simulink model "mechanics_sensor"  (R2014a)
settings: Solver=ode45  StartTime=0.0  StopTime=10.0  RelTol=1e-3
values from neighbouring files (symbols this model uses):
  c = [x y z]'    [estimation_initfcn.m]
  I_xx = 1/12*m*(y^2+z^2)    (= 0.00181666666667)    [estimation_initfcn.m]
  I_yy = 1/12*m*(x^2+z^2)    (= 0.0418166666667)    [estimation_initfcn.m]
  I_zz = 1/12*m*(y^2+x^2)    (= 0.0433333333333)    [estimation_initfcn.m]
  m = 2    [estimation_initfcn.m]
  x = 0.5    [estimation_initfcn.m]
  y = 0.1    [estimation_initfcn.m]
  z = 0.03    [estimation_initfcn.m]
undefined symbols (not defined in the file or in its folder): X, Y, Z
libraries: nesl_utility x53, sm_lib x11, aerolibutil x6
settings Model: Creator=wirnshofer  LastModifiedBy=wirnshofer

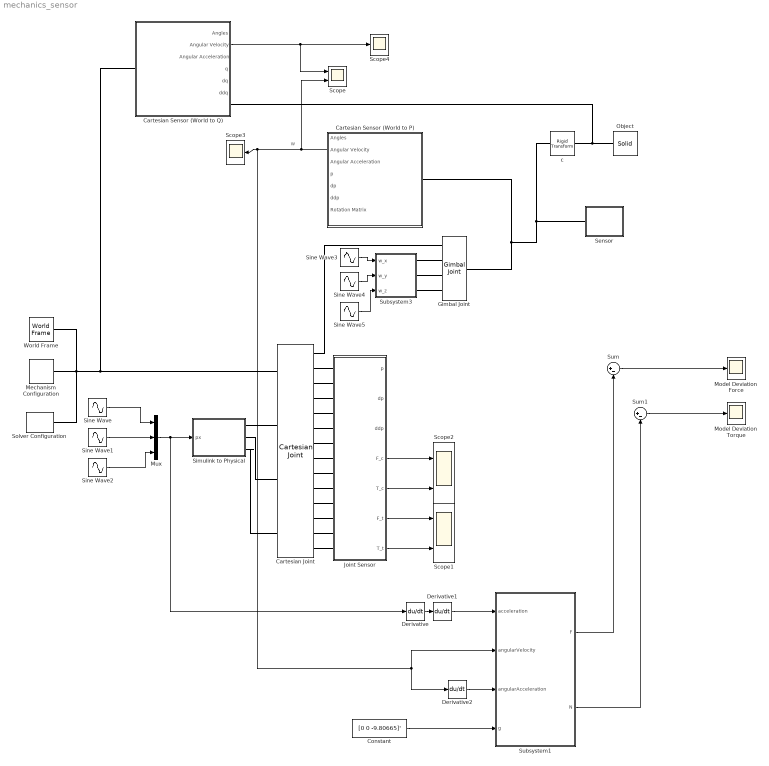
== system mechanics_sensor ==
  note: w
  Cartesian Joint : sm_lib/Joints/Cartesian Joint  SenseConstraintForce=on  SenseConstraintForceX=off  SenseConstraintForceY=off  SenseConstraintForceZ=off  SenseConstraintTorque=on  SenseConstraintTorqueX=off  SenseConstraintTorqueY=off  SenseConstraintTorqueZ=off  SenseTotalForce=on  SenseTotalForceX=off  SenseTotalForceY=off  SenseTotalForceZ=off  SenseTotalTorque=on  SenseTotalTorqueX=off  SenseTotalTorqueY=off  SenseTotalTorqueZ=off  CompositeWrenchDir=FollowerOnBase  CompositeWrenchFrame=BaseFrame  PxEquilibriumPosition=0  PxEquilibriumPositionUnits=m  PxSpringStiffness=0  PxSpringStiffnessUnits=N/m  PxDampingCoefficient=0  PxDampingCoefficientUnits=N/(m/s)  PxTorqueActuationMode=ComputedTorque  PxMotionActuationMode=InputMotion  PxSensePosition=on  PxSenseVelocity=on  PxSenseAcceleration=on  PxSenseTorqueForce=off  PxPositionTargetValue=0  PxPositionTargetValueUnits=m  PxPositionTargetSpecify=off  PxPositionTargetPriority=High  PxVelocityTargetValue=0  PxVelocityTargetValueUnits=m/s  PxVelocityTargetSpecify=off  PxVelocityTargetPriority=High  PyEquilibriumPosition=0  PyEquilibriumPositionUnits=m  PySpringStiffness=0  PySpringStiffnessUnits=N/m  PyDampingCoefficient=0  PyDampingCoefficientUnits=N/(m/s)  PyTorqueActuationMode=ComputedTorque  PyMotionActuationMode=InputMotion  PySensePosition=on  PySenseVelocity=on  PySenseAcceleration=on  PySenseTorqueForce=off  PyPositionTargetValue=0  PyPositionTargetValueUnits=m  PyPositionTargetSpecify=off  PyPositionTargetPriority=High  PyVelocityTargetValue=0  PyVelocityTargetValueUnits=m/s  PyVelocityTargetSpecify=off  PyVelocityTargetPriority=High  PzEquilibriumPosition=0  PzEquilibriumPositionUnits=m  PzSpringStiffness=0  PzSpringStiffnessUnits=N/m  PzDampingCoefficient=0  PzDampingCoefficientUnits=N/(m/s)  PzTorqueActuationMode=ComputedTorque  PzMotionActuationMode=InputMotion  PzSensePosition=on  PzSenseVelocity=on  PzSenseAcceleration=on  PzSenseTorqueForce=off  PzPositionTargetValue=0  PzPositionTargetValueUnits=m  PzPositionTargetSpecify=off  PzPositionTargetPriority=High  PzVelocityTargetValue=0  PzVelocityTargetValueUnits=m/s  PzVelocityTargetSpecify=off  PzVelocityTargetPriority=High  BlockFunction=simmechanics.library.joints.cartesian_joint
  Cartesian Sensor (World to P) : Subsystem
  Cartesian Sensor (World to Q) : Subsystem
  Constant : Constant  Value=[0 0 -9.80665]'
  Derivative : Derivative
  Derivative1 : Derivative
  Derivative2 : Derivative
  Gimbal Joint : sm_lib/Joints/Gimbal Joint  SenseConstraintForce=off  SenseConstraintForceX=off  SenseConstraintForceY=off  SenseConstraintForceZ=off  SenseConstraintTorque=off  SenseConstraintTorqueX=off  SenseConstraintTorqueY=off  SenseConstraintTorqueZ=off  SenseTotalForce=off  SenseTotalForceX=off  SenseTotalForceY=off  SenseTotalForceZ=off  SenseTotalTorque=off  SenseTotalTorqueX=off  SenseTotalTorqueY=off  SenseTotalTorqueZ=off  CompositeWrenchDir=FollowerOnBase  CompositeWrenchFrame=BaseFrame  RxEquilibriumPosition=0  RxEquilibriumPositionUnits=deg  RxSpringStiffness=0  RxSpringStiffnessUnits=N*m/deg  RxDampingCoefficient=0  RxDampingCoefficientUnits=N*m/(deg/s)  RxTorqueActuationMode=ComputedTorque  RxMotionActuationMode=InputMotion  RxSensePosition=off  RxSenseVelocity=off  RxSenseAcceleration=off  RxSenseTorqueForce=off  RxPositionTargetValue=0  RxPositionTargetValueUnits=deg  RxPositionTargetSpecify=off  RxPositionTargetPriority=High  RxVelocityTargetValue=0  RxVelocityTargetValueUnits=deg/s  RxVelocityTargetSpecify=off  RxVelocityTargetPriority=High  RyEquilibriumPosition=0  RyEquilibriumPositionUnits=deg  RySpringStiffness=0  RySpringStiffnessUnits=N*m/deg  RyDampingCoefficient=0  RyDampingCoefficientUnits=N*m/(deg/s)  RyTorqueActuationMode=ComputedTorque  RyMotionActuationMode=InputMotion  RySensePosition=off  RySenseVelocity=off  RySenseAcceleration=off  RySenseTorqueForce=off  RyPositionTargetValue=0  RyPositionTargetValueUnits=deg  RyPositionTargetSpecify=off  RyPositionTargetPriority=High  RyVelocityTargetValue=0  RyVelocityTargetValueUnits=deg/s  RyVelocityTargetSpecify=off  RyVelocityTargetPriority=High  RzEquilibriumPosition=0  RzEquilibriumPositionUnits=deg  RzSpringStiffness=0  RzSpringStiffnessUnits=N*m/deg  RzDampingCoefficient=0  RzDampingCoefficientUnits=N*m/(deg/s)  RzTorqueActuationMode=ComputedTorque  RzMotionActuationMode=InputMotion  RzSensePosition=off  RzSenseVelocity=off  RzSenseAcceleration=off  RzSenseTorqueForce=off  RzPositionTargetValue=0  RzPositionTargetValueUnits=deg  RzPositionTargetSpecify=off  RzPositionTargetPriority=High  RzVelocityTargetValue=0  RzVelocityTargetValueUnits=deg/s  RzVelocityTargetSpecify=off  RzVelocityTargetPriority=High  BlockFunction=simmechanics.library.joints.gimbal_joint
  Joint Sensor : Subsystem
  Mechanism Configuration : sm_lib/Utilities/Mechanism Configuration  UniformGravity=Constant  GravityVector=[0 0 -9.80665]  GravityUnits=m/s^2  LinearizationDelta=0.001  BlockFunction=simmechanics.library.utilities.mechanism_configuration
  Model Deviation Force : Scope
      settings: TimeRange=10  YMin=-1.3  YMax=0.8  SaveName=modelDeviationForce
  Model Deviation Torque : Scope
      settings: TimeRange=10  YMin=-1.3  YMax=0.8  SaveName=modelDeviationForce1
  Mux : Mux  Inputs=3
  Object : sm_lib/Body Elements/Solid  InertiaType=Custom  Mass=m  MassUnits=kg  CenterOfMass=[0 0 0]  CenterOfMassUnits=m  MomentsOfInertia=[I_xx I_yy I_zz]  MomentsOfInertiaUnits=kg*m^2  ProductsOfInertia=[0 0 0]  ProductsOfInertiaUnits=kg*m^2  DensityBased=on  Density=1000  DensityUnits=kg/(m^3)  GraphicType=FromGeometry  MarkerShape=Sphere  MarkerSize=10  MarkerSizeUnits=m  GraphicVisPropType=SimpleVisualProperties  GraphicDiffuseColor=[0.5 0.5 0.5]  GraphicSpecularColor=[0.5 0.5 0.5 1.0]  GraphicAmbientColor=[0.15 0.15 0.15 1.0]  GraphicEmissiveColor=[0.0 0.0 0.0 1.0]  GraphicShininess=75  GraphicOpacity=1.0  GeometryShape=Brick  RectangleSize=[1 1]  RectangleSizeUnits=m  BrickDimensions=[x y z]  BrickDimensionUnits=m  CylinderRadius=1  CylinderRadiusUnits=m  CylinderLength=1  CylinderLengthUnits=m  SphereRadius=1  SphereRadiusUnits=m  EllipsoidRadii=[1 1 1]  EllipsoidRadiiUnits=m  ExtrusionCrossSection=[1 1; -1 1; -1 -1; 1 -1]  ExtrusionCrossSectionUnits=m  ExtrusionLength=1  ExtrusionLengthUnits=m  PolygonNumSides=3  PolygonOuterRadius=1  PolygonOuterRadiusUnits=m  ExtGeomFileType=STL  ExtGeomFileUnits=m  RevolutionCrossSection=[1 1; 1 -1; 2 -1; 2 1]  RevolutionCrossSectionUnits=m  RevolutionExtent=Full  RevolutionAngle=180  RevolutionAngleUnits=deg  BlockFunction=simmechanics.library.body_elements.solid
  Scope : Scope  NumInputPorts=2
      settings: YMin=-0.3~-0.3  YMax=0.5~0.3
  Scope1 : Scope  NumInputPorts=2
      settings: TimeRange=10  YMin=-1.146992373051417~-500  YMax=1.739930939930119~500
  Scope2 : Scope  NumInputPorts=2
      settings: TimeRange=10  YMin=-1.146992373051417~-500  YMax=1.739930939930119~500  SaveName=ScopeData2
  Scope3 : Scope
      settings: YMin=-0.3  YMax=0.5  SaveName=ScopeData3
  Scope4 : Scope
      settings: YMin=-0.3  YMax=0.5  SaveName=ScopeData4
  Sensor : Subsystem
  Simulink to Physical : Subsystem
  Sine Wave : Sin  Amplitude=0.2  Frequency=7  SampleTime=0
  Sine Wave1 : Sin  Amplitude=0.3  Frequency=4  SampleTime=0
  Sine Wave2 : Sin  Amplitude=0.2  Frequency=10  SampleTime=0
  Sine Wave3 : Sin  Amplitude=0.5  Frequency=10  SampleTime=0
  Sine Wave4 : Sin  Amplitude=0.6  Frequency=8  SampleTime=0
  Sine Wave5 : Sin  Frequency=7  SampleTime=0
  Solver Configuration : nesl_utility/Solver Configuration  PhysicalDomain=network_engine_domain  SubClassName=solver  LeftPortType=input  RightPortType=generic  Accelerate=off  Tones=[]  Harmonics=[]  SimulateNoise=off  Profile=off  UseLocalSampling=off  EnableSwitchedLinearOptims=on  FrequencyDomain=off  UseCCode=off  RelTol=0.001  AbsTol=1e-06  MinStep=1e-09  ToWorkspace=off  DoDC=off  ResidualTolerance=1e-09  UseLocalSolver=off  LocalSolverChoice=NE_BACKWARD_EULER_ADVANCER  LocalSolverSampleTime=0.001  DoFixedCost=off  MaxNonlinIter=3  MaxModeIter=2  LinearAlgebra=Sparse  DelaysMemoryBudget=1024  AutomaticFiltering=on  FilteringTimeConstant=0.001
  Subsystem1 : Subsystem
  Subsystem3 : Subsystem
  Sum : Sum  Inputs=|+-
  Sum1 : Sum  Inputs=|+-
  World Frame : sm_lib/Frames and Transforms/World Frame  BlockFunction=simmechanics.library.frames_transforms.world_frame
  c : sm_lib/Frames and Transforms/Rigid Transform  TranslationMethod=Cartesian  TranslationLengthUnit=m  TranslationStandardAxis=+Z  TranslationStandardOffset=0  TranslationCartesianOffset=c  TranslationROffset=0  TranslationROffsetUnits=m  TranslationZOffset=0  TranslationZOffsetUnits=m  TranslationThetaOffset=0  TranslationThetaOffsetUnits=deg  RotationMethod=None  RotationAngleUnits=deg  RotationStandardAxis=+Z  RotationAngle=0  RotationArbitraryAxis=[0 0 1]  FollAlignAxisA=+X  BaseAlignAxisA=+Y  FollAlignAxisB=+Y  BaseAlignAxisB=+Z  BlockFunction=simmechanics.library.frames_transforms.rigid_transform
  wires:
  Sine Wave/1 -> Mux/1
  Sine Wave1/1 -> Mux/2
  Sine Wave2/1 -> Mux/3
  Joint Sensor/6(F_t) -> Scope1/1
  Joint Sensor/7(T_t) -> Scope1/2
  Joint Sensor/4(F_c) -> Scope2/1
  Joint Sensor/5(T_c) -> Scope2/2
  Cartesian Sensor (World to P)/2(Angular Velocity) -> Derivative2/1, Subsystem1/2(angularVelocity), Scope3/1, Scope/2
  Cartesian Sensor (World to Q)/2(Angular Velocity) -> Scope/1, Scope4/1
  Sine Wave3/1 -> Subsystem3/1(w_x)
  Sine Wave4/1 -> Subsystem3/2(w_y)
  Sine Wave5/1 -> Subsystem3/3(w_z)
  Mux/1 -> Derivative/1, Simulink to Physical/1(px)
  Derivative/1 -> Derivative1/1
  Derivative1/1 -> Subsystem1/1(acceleration)
  Derivative2/1 -> Subsystem1/3(angularAcceleration)
  Constant/1 -> Subsystem1/4(g)
  ? -> Sum/1
  Sum/1 -> Model Deviation Force/1
  ? -> Sum1/1
  Subsystem1/1(F) -> Sum/2
  Subsystem1/2(N) -> Sum1/2
  Sum1/1 -> Model Deviation Torque/1
  connections:
  Cartesian Sensor (World to Q)/RConn1 -- Object/RConn1 -- c/RConn1
  Solver Configuration/RConn1 -- World Frame/RConn1 -- Cartesian Joint/LConn1 -- Cartesian Sensor (World to Q)/LConn1 -- Mechanism Configuration/RConn1
  Gimbal Joint/RConn1 -- Cartesian Sensor (World to P)/LConn1 -- Sensor/RConn1 -- c/LConn1
  Simulink to Physical/RConn1 -- Cartesian Joint/LConn2
  Simulink to Physical/RConn2 -- Cartesian Joint/LConn3
  Simulink to Physical/RConn3 -- Cartesian Joint/LConn4
  Joint Sensor/LConn1 -- Cartesian Joint/RConn2
  Joint Sensor/LConn2 -- Cartesian Joint/RConn3
  Joint Sensor/LConn3 -- Cartesian Joint/RConn4
  Joint Sensor/LConn4 -- Cartesian Joint/RConn5
  Joint Sensor/LConn5 -- Cartesian Joint/RConn6
  Joint Sensor/LConn6 -- Cartesian Joint/RConn7
  Joint Sensor/LConn8 -- Cartesian Joint/RConn9
  Joint Sensor/LConn9 -- Cartesian Joint/RConn10
  Joint Sensor/LConn10 -- Cartesian Joint/RConn11
  Joint Sensor/LConn11 -- Cartesian Joint/RConn12
  Joint Sensor/LConn12 -- Cartesian Joint/RConn13
  Joint Sensor/LConn13 -- Cartesian Joint/RConn14
  Subsystem3/RConn1 -- Gimbal Joint/LConn2
  Subsystem3/RConn2 -- Gimbal Joint/LConn3
  Joint Sensor/LConn7 -- Cartesian Joint/RConn8
  Subsystem3/RConn3 -- Gimbal Joint/LConn4
  Cartesian Joint/RConn1 -- Gimbal Joint/LConn1

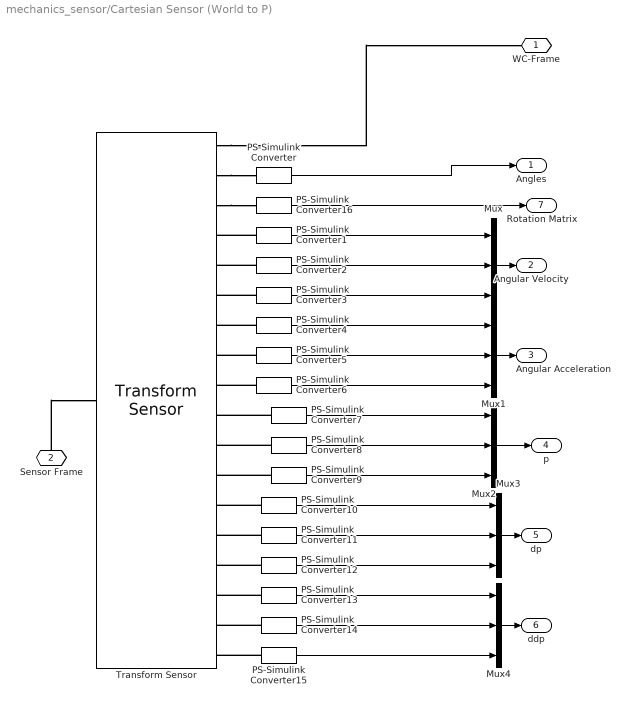
== system mechanics_sensor/Cartesian Sensor (World to P) ==
  Mux{,1..4} (5 alike) : Mux  Inputs=3
  PS-Simulink Converter{,1..16} (17 alike) : nesl_utility/PS-Simulink Converter  PhysicalDomain=network_engine_domain  SubClassName=ps_output  LeftPortType=input  RightPortType=output  PseudoPeriodic=off  Frequencies=[]  Unit=1  AffineConversion=off
  Transform Sensor : sm_lib/Frames and Transforms/Transform Sensor  MeasurementFrame=World  SenseAngle=on  SenseAxis=off  SenseAngle1=off  SenseAngle2=off  SenseAngle3=off  SenseQ=off  SenseR=on  SenseOmegaX=on  SenseOmegaY=on  SenseOmegaZ=on  SenseOmega1=off  SenseOmega2=off  SenseOmega3=off  SenseQDot=off  SenseRDot=off  SenseAlphaX=on  SenseAlphaY=on  SenseAlphaZ=on  SenseAlpha1=off  SenseAlpha2=off  SenseAlpha3=off  SenseQDDot=off  SenseRDDot=off  SenseX=on  SenseY=on  SenseZ=on  SenseRad=off  SenseAzim=off  SenseDist=off  SenseInc=off  SenseXDot=on  SenseYDot=on  SenseZDot=on  SenseRadDot=off  SenseAzimDot=off  SenseDistDot=off  SenseIncDot=off  SenseXDDot=on  SenseYDDot=on  SenseZDDot=on  SenseRadDDot=off  SenseAzimDDot=off  SenseDistDDot=off  SenseIncDDot=off  BlockFunction=simmechanics.library.frames_transforms.transform_sensor
  WC-Frame : PMIOPort  Port=1  Side=Right
  Sensor Frame : PMIOPort  Port=2  Side=Left
  Angles : Outport
  Angular Velocity : Outport  Port=2
  Angular Acceleration : Outport  Port=3
  p : Outport  Port=4
  dp : Outport  Port=5
  ddp : Outport  Port=6
  Rotation Matrix : Outport  Port=7
  wires:
  PS-Simulink Converter2/1 -> Mux/2
  PS-Simulink Converter5/1 -> Mux1/2
  Mux1/1 -> Angular Acceleration/1
  PS-Simulink Converter1/1 -> Mux/1
  Mux/1 -> Angular Velocity/1
  PS-Simulink Converter6/1 -> Mux1/3
  PS-Simulink Converter/1 -> Angles/1
  PS-Simulink Converter3/1 -> Mux/3
  PS-Simulink Converter4/1 -> Mux1/1
  PS-Simulink Converter8/1 -> Mux2/2
  Mux2/1 -> p/1
  PS-Simulink Converter9/1 -> Mux2/3
  PS-Simulink Converter7/1 -> Mux2/1
  PS-Simulink Converter11/1 -> Mux3/2
  Mux3/1 -> dp/1
  PS-Simulink Converter12/1 -> Mux3/3
  PS-Simulink Converter10/1 -> Mux3/1
  PS-Simulink Converter14/1 -> Mux4/2
  Mux4/1 -> ddp/1
  PS-Simulink Converter15/1 -> Mux4/3
  PS-Simulink Converter13/1 -> Mux4/1
  PS-Simulink Converter16/1 -> Rotation Matrix/1
  connections:
  Transform Sensor/RConn1 -- WC-Frame/RConn1
  Sensor Frame/RConn1 -- Transform Sensor/LConn1
  Transform Sensor/RConn2 -- PS-Simulink Converter/LConn1
  PS-Simulink Converter6/LConn1 -- Transform Sensor/RConn9
  PS-Simulink Converter2/LConn1 -- Transform Sensor/RConn5
  PS-Simulink Converter5/LConn1 -- Transform Sensor/RConn8
  PS-Simulink Converter1/LConn1 -- Transform Sensor/RConn4
  PS-Simulink Converter4/LConn1 -- Transform Sensor/RConn7
  PS-Simulink Converter3/LConn1 -- Transform Sensor/RConn6
  PS-Simulink Converter14/LConn1 -- Transform Sensor/RConn17
  PS-Simulink Converter10/LConn1 -- Transform Sensor/RConn13
  PS-Simulink Converter13/LConn1 -- Transform Sensor/RConn16
  PS-Simulink Converter12/LConn1 -- Transform Sensor/RConn15
  PS-Simulink Converter11/LConn1 -- Transform Sensor/RConn14
  PS-Simulink Converter15/LConn1 -- Transform Sensor/RConn18
  PS-Simulink Converter8/LConn1 -- Transform Sensor/RConn11
  PS-Simulink Converter9/LConn1 -- Transform Sensor/RConn12
  PS-Simulink Converter7/LConn1 -- Transform Sensor/RConn10
  Transform Sensor/RConn3 -- PS-Simulink Converter16/LConn1

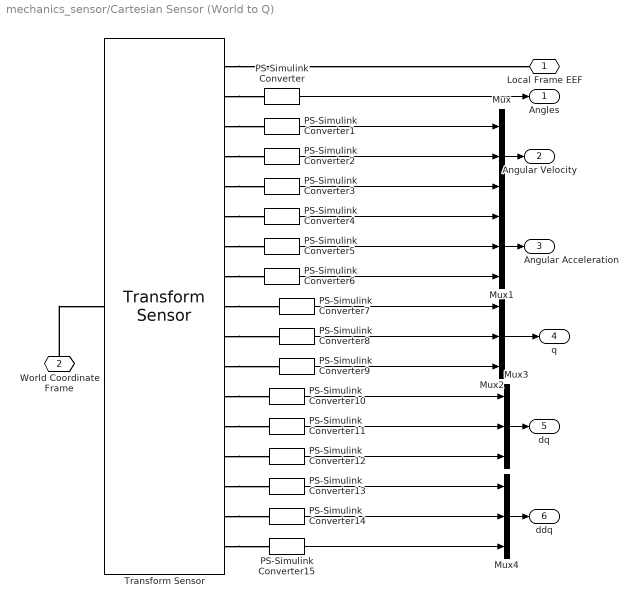
== system mechanics_sensor/Cartesian Sensor (World to Q) ==
  Mux{,1..4} (5 alike) : Mux  Inputs=3
  PS-Simulink Converter{,1..15} (16 alike) : nesl_utility/PS-Simulink Converter  PhysicalDomain=network_engine_domain  SubClassName=ps_output  LeftPortType=input  RightPortType=output  PseudoPeriodic=off  Frequencies=[]  Unit=1  AffineConversion=off
  Transform Sensor : sm_lib/Frames and Transforms/Transform Sensor  MeasurementFrame=World  SenseAngle=on  SenseAxis=off  SenseAngle1=off  SenseAngle2=off  SenseAngle3=off  SenseQ=off  SenseR=off  SenseOmegaX=on  SenseOmegaY=on  SenseOmegaZ=on  SenseOmega1=off  SenseOmega2=off  SenseOmega3=off  SenseQDot=off  SenseRDot=off  SenseAlphaX=on  SenseAlphaY=on  SenseAlphaZ=on  SenseAlpha1=off  SenseAlpha2=off  SenseAlpha3=off  SenseQDDot=off  SenseRDDot=off  SenseX=on  SenseY=on  SenseZ=on  SenseRad=off  SenseAzim=off  SenseDist=off  SenseInc=off  SenseXDot=on  SenseYDot=on  SenseZDot=on  SenseRadDot=off  SenseAzimDot=off  SenseDistDot=off  SenseIncDot=off  SenseXDDot=on  SenseYDDot=on  SenseZDDot=on  SenseRadDDot=off  SenseAzimDDot=off  SenseDistDDot=off  SenseIncDDot=off  BlockFunction=simmechanics.library.frames_transforms.transform_sensor
  Local Frame EEF : PMIOPort  Port=1  Side=Right
  World Coordinate Frame : PMIOPort  Port=2  Side=Left
  Angles : Outport
  Angular Velocity : Outport  Port=2
  Angular Acceleration : Outport  Port=3
  q : Outport  Port=4
  dq : Outport  Port=5
  ddq : Outport  Port=6
  wires:
  PS-Simulink Converter2/1 -> Mux/2
  PS-Simulink Converter5/1 -> Mux1/2
  Mux1/1 -> Angular Acceleration/1
  PS-Simulink Converter1/1 -> Mux/1
  Mux/1 -> Angular Velocity/1
  PS-Simulink Converter6/1 -> Mux1/3
  PS-Simulink Converter/1 -> Angles/1
  PS-Simulink Converter3/1 -> Mux/3
  PS-Simulink Converter4/1 -> Mux1/1
  PS-Simulink Converter8/1 -> Mux2/2
  Mux2/1 -> q/1
  PS-Simulink Converter9/1 -> Mux2/3
  PS-Simulink Converter7/1 -> Mux2/1
  PS-Simulink Converter11/1 -> Mux3/2
  Mux3/1 -> dq/1
  PS-Simulink Converter12/1 -> Mux3/3
  PS-Simulink Converter10/1 -> Mux3/1
  PS-Simulink Converter14/1 -> Mux4/2
  Mux4/1 -> ddq/1
  PS-Simulink Converter15/1 -> Mux4/3
  PS-Simulink Converter13/1 -> Mux4/1
  connections:
  Transform Sensor/RConn7 -- PS-Simulink Converter5/LConn1
  Transform Sensor/RConn1 -- Local Frame EEF/RConn1
  Transform Sensor/RConn5 -- PS-Simulink Converter3/LConn1
  Transform Sensor/RConn8 -- PS-Simulink Converter6/LConn1
  Transform Sensor/RConn3 -- PS-Simulink Converter1/LConn1
  Transform Sensor/RConn6 -- PS-Simulink Converter4/LConn1
  World Coordinate Frame/RConn1 -- Transform Sensor/LConn1
  Transform Sensor/RConn4 -- PS-Simulink Converter2/LConn1
  Transform Sensor/RConn2 -- PS-Simulink Converter/LConn1
  Transform Sensor/RConn9 -- PS-Simulink Converter7/LConn1
  Transform Sensor/RConn10 -- PS-Simulink Converter8/LConn1
  Transform Sensor/RConn11 -- PS-Simulink Converter9/LConn1
  Transform Sensor/RConn12 -- PS-Simulink Converter10/LConn1
  Transform Sensor/RConn13 -- PS-Simulink Converter11/LConn1
  Transform Sensor/RConn14 -- PS-Simulink Converter12/LConn1
  Transform Sensor/RConn15 -- PS-Simulink Converter13/LConn1
  Transform Sensor/RConn16 -- PS-Simulink Converter14/LConn1
  Transform Sensor/RConn17 -- PS-Simulink Converter15/LConn1

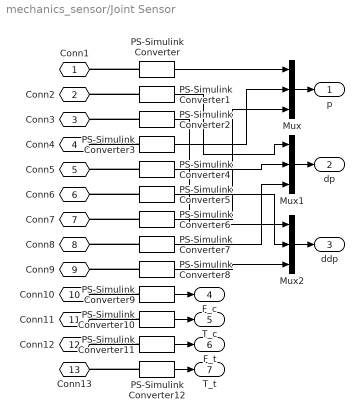
== system mechanics_sensor/Joint Sensor ==
  Mux : Mux  Inputs=3
  Mux1 : Mux  Inputs=3
  Mux2 : Mux  Inputs=3
  PS-Simulink Converter{,1..12} (13 alike) : nesl_utility/PS-Simulink Converter  PhysicalDomain=network_engine_domain  SubClassName=ps_output  LeftPortType=input  RightPortType=output  PseudoPeriodic=off  Frequencies=[]  Unit=1  AffineConversion=off
  Conn1 : PMIOPort  Port=1  Side=Left
  Conn2 : PMIOPort  Port=2  Side=Left
  Conn3 : PMIOPort  Port=3  Side=Left
  Conn4 : PMIOPort  Port=4  Side=Left
  Conn5 : PMIOPort  Port=5  Side=Left
  Conn6 : PMIOPort  Port=6  Side=Left
  Conn7 : PMIOPort  Port=7  Side=Left
  Conn8 : PMIOPort  Port=8  Side=Left
  Conn9 : PMIOPort  Port=9  Side=Left
  Conn10 : PMIOPort  Port=10  Side=Left
  Conn11 : PMIOPort  Port=11  Side=Left
  Conn12 : PMIOPort  Port=12  Side=Left
  Conn13 : PMIOPort  Port=13  Side=Left
  p : Outport
  dp : Outport  Port=2
  ddp : Outport  Port=3
  F_c : Outport  Port=4
  T_c : Outport  Port=5
  F_t : Outport  Port=6
  T_t : Outport  Port=7
  wires:
  PS-Simulink Converter5/1 -> Mux2/2
  PS-Simulink Converter/1 -> Mux/1
  PS-Simulink Converter3/1 -> Mux/2
  Mux1/1 -> dp/1
  Mux2/1 -> ddp/1
  Mux/1 -> p/1
  PS-Simulink Converter6/1 -> Mux/3
  PS-Simulink Converter4/1 -> Mux1/2
  PS-Simulink Converter1/1 -> Mux1/1
  PS-Simulink Converter11/1 -> F_t/1
  PS-Simulink Converter7/1 -> Mux1/3
  PS-Simulink Converter12/1 -> T_t/1
  PS-Simulink Converter2/1 -> Mux2/1
  PS-Simulink Converter8/1 -> Mux2/3
  PS-Simulink Converter9/1 -> F_c/1
  PS-Simulink Converter10/1 -> T_c/1
  connections:
  PS-Simulink Converter9/LConn1 -- Conn10/RConn1
  PS-Simulink Converter7/LConn1 -- Conn8/RConn1
  PS-Simulink Converter10/LConn1 -- Conn11/RConn1
  PS-Simulink Converter6/LConn1 -- Conn7/RConn1
  PS-Simulink Converter4/LConn1 -- Conn5/RConn1
  PS-Simulink Converter12/LConn1 -- Conn13/RConn1
  PS-Simulink Converter8/LConn1 -- Conn9/RConn1
  PS-Simulink Converter/LConn1 -- Conn1/RConn1
  PS-Simulink Converter2/LConn1 -- Conn3/RConn1
  PS-Simulink Converter5/LConn1 -- Conn6/RConn1
  PS-Simulink Converter3/LConn1 -- Conn4/RConn1
  PS-Simulink Converter11/LConn1 -- Conn12/RConn1
  PS-Simulink Converter1/LConn1 -- Conn2/RConn1

== system mechanics_sensor/Sensor ==
  Solid : sm_lib/Body Elements/Solid  InertiaType=CalculateFromGeometry  Mass=0.000000000001  MassUnits=kg  CenterOfMass=[0 0 0]  CenterOfMassUnits=m  MomentsOfInertia=[1 1 1]  MomentsOfInertiaUnits=kg*m^2  ProductsOfInertia=[0 0 0]  ProductsOfInertiaUnits=kg*m^2  DensityBased=off  Density=1000  DensityUnits=kg/(m^3)  GraphicType=FromGeometry  MarkerShape=Sphere  MarkerSize=10  MarkerSizeUnits=m  GraphicVisPropType=SimpleVisualProperties  GraphicDiffuseColor=[0.0 0.0 1.0]  GraphicSpecularColor=[0.5 0.5 0.5 1.0]  GraphicAmbientColor=[0.15 0.15 0.15 1.0]  GraphicEmissiveColor=[0.0 0.0 0.0 1.0]  GraphicShininess=75  GraphicOpacity=1.0  GeometryShape=Cylinder  RectangleSize=[1 1]  RectangleSizeUnits=m  BrickDimensions=[1 1 1]  BrickDimensionUnits=m  CylinderRadius=0.025  CylinderRadiusUnits=m  CylinderLength=0.03  CylinderLengthUnits=m  SphereRadius=1  SphereRadiusUnits=m  EllipsoidRadii=[1 1 1]  EllipsoidRadiiUnits=m  ExtrusionCrossSection=[1 1; -1 1; -1 -1; 1 -1]  ExtrusionCrossSectionUnits=m  ExtrusionLength=1  ExtrusionLengthUnits=m  PolygonNumSides=3  PolygonOuterRadius=1  PolygonOuterRadiusUnits=m  ExtGeomFileType=STL  ExtGeomFileUnits=m  RevolutionCrossSection=[1 1; 1 -1; 2 -1; 2 1]  RevolutionCrossSectionUnits=m  RevolutionExtent=Full  RevolutionAngle=180  RevolutionAngleUnits=deg  BlockFunction=simmechanics.library.body_elements.solid
  Transform5 : sm_lib/Frames and Transforms/Rigid Transform  TranslationMethod=None  TranslationLengthUnit=mm  TranslationStandardAxis=+Z  TranslationStandardOffset=0  TranslationCartesianOffset=[0 0 0]  TranslationROffset=0  TranslationROffsetUnits=m  TranslationZOffset=0  TranslationZOffsetUnits=m  TranslationThetaOffset=0  TranslationThetaOffsetUnits=deg  RotationMethod=StandardAxis  RotationAngleUnits=deg  RotationStandardAxis=+Y  RotationAngle=90  RotationArbitraryAxis=[0 0 1]  FollAlignAxisA=+X  BaseAlignAxisA=+Y  FollAlignAxisB=+Y  BaseAlignAxisB=+Z  BlockFunction=simmechanics.library.frames_transforms.rigid_transform
  Transform6 : sm_lib/Frames and Transforms/Rigid Transform  TranslationMethod=Cartesian  TranslationLengthUnit=m  TranslationStandardAxis=+Z  TranslationStandardOffset=0  TranslationCartesianOffset=[0.015 0 0]  TranslationROffset=0  TranslationROffsetUnits=m  TranslationZOffset=0  TranslationZOffsetUnits=m  TranslationThetaOffset=0  TranslationThetaOffsetUnits=deg  RotationMethod=None  RotationAngleUnits=deg  RotationStandardAxis=+Z  RotationAngle=0  RotationArbitraryAxis=[0 0 1]  FollAlignAxisA=+X  BaseAlignAxisA=+Y  FollAlignAxisB=+Y  BaseAlignAxisB=+Z  BlockFunction=simmechanics.library.frames_transforms.rigid_transform
  Conn2 : PMIOPort  Port=1  Side=Right
  connections:
  Transform5/LConn1 -- Solid/RConn1
  Transform6/RConn1 -- Conn2/RConn1
  Transform5/RConn1 -- Transform6/LConn1

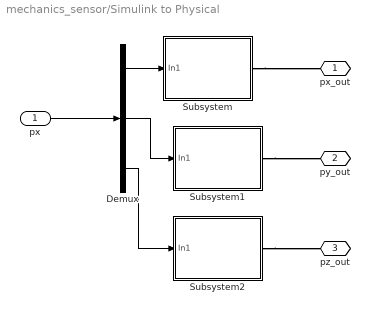
== system mechanics_sensor/Simulink to Physical ==
  px : Inport
  Demux : Demux  Outputs=3
  Subsystem : Subsystem
  Subsystem1 : Subsystem
  Subsystem2 : Subsystem
  px_out : PMIOPort  Port=1  Side=Right
  py_out : PMIOPort  Port=2  Side=Right
  pz_out : PMIOPort  Port=3  Side=Right
  wires:
  px/1 -> Demux/1
  Demux/1 -> Subsystem/1(In1)
  Demux/2 -> Subsystem1/1(In1)
  Demux/3 -> Subsystem2/1(In1)
  connections:
  Subsystem2/RConn1 -- pz_out/RConn1
  Subsystem/RConn1 -- px_out/RConn1
  Subsystem1/RConn1 -- py_out/RConn1

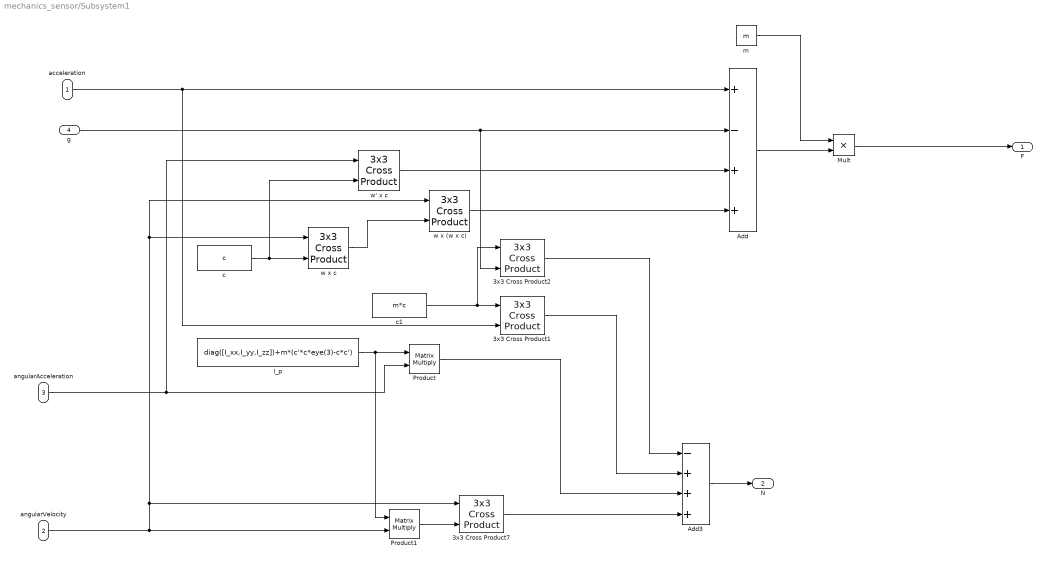
== system mechanics_sensor/Subsystem1 ==
  acceleration : Inport
  angularVelocity : Inport  Port=2
  angularAcceleration : Inport  Port=3
  g : Inport  Port=4
  3x3 Cross Product1 : aerolibutil/3x3 Cross Product
  3x3 Cross Product2 : aerolibutil/3x3 Cross Product
  3x3 Cross Product7 : aerolibutil/3x3 Cross Product
  Add : Sum  Inputs=+-++
  Add3 : Sum  Inputs=-+++
  I_p : Constant  Value=diag([I_xx,I_yy,I_zz])+m*(c'*c*eye(3)-c*c')  VectorParams1D=off
  Mult : Product  Inputs=**
  Product : Product  Multiplication=Matrix(*)
  Product1 : Product  Multiplication=Matrix(*)
  c : Constant  Value=c
  c1 : Constant  Value=m*c
  m : Constant  Value=m
  w x (w x c) : aerolibutil/3x3 Cross Product
  w x c : aerolibutil/3x3 Cross Product
  w' x c : aerolibutil/3x3 Cross Product
  F : Outport
  N : Outport  Port=2
  wires:
  acceleration/1 -> 3x3 Cross Product1/2, Add/1
  angularVelocity/1 -> w x (w x c)/1, w x c/1, 3x3 Cross Product7/1, Product1/2
  angularAcceleration/1 -> Product/2, w' x c/1
  Product1/1 -> 3x3 Cross Product7/2
  Mult/1 -> F/1
  m/1 -> Mult/1
  w' x c/1 -> Add/3
  w x c/1 -> w x (w x c)/2
  w x (w x c)/1 -> Add/4
  3x3 Cross Product7/1 -> Add3/4
  Add/1 -> Mult/2
  g/1 -> 3x3 Cross Product2/2, Add/2
  c/1 -> w' x c/2, w x c/2
  I_p/1 -> Product1/1, Product/1
  c1/1 -> 3x3 Cross Product2/1, 3x3 Cross Product1/1
  3x3 Cross Product1/1 -> Add3/2
  3x3 Cross Product2/1 -> Add3/1
  Add3/1 -> N/1
  Product/1 -> Add3/3

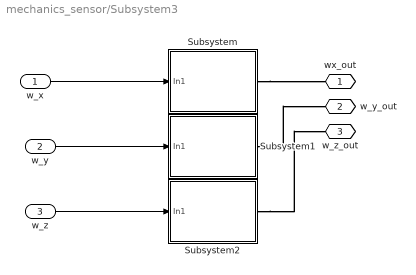
== system mechanics_sensor/Subsystem3 ==
  w_x : Inport
  w_y : Inport  Port=2
  w_z : Inport  Port=3
  Subsystem : Subsystem
  Subsystem1 : Subsystem
  Subsystem2 : Subsystem
  wx_out : PMIOPort  Port=1  Side=Right
  w_y_out : PMIOPort  Port=2  Side=Right
  w_z_out : PMIOPort  Port=3  Side=Right
  wires:
  w_z/1 -> Subsystem2/1(In1)
  w_y/1 -> Subsystem1/1(In1)
  w_x/1 -> Subsystem/1(In1)
  connections:
  Subsystem1/RConn1 -- w_y_out/RConn1
  Subsystem/RConn1 -- wx_out/RConn1
  Subsystem2/RConn1 -- w_z_out/RConn1

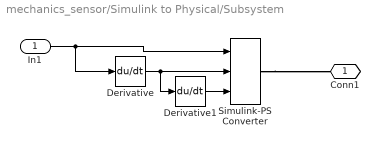
== system mechanics_sensor/Simulink to Physical/Subsystem ==
  In1 : Inport
  Derivative : Derivative
  Derivative1 : Derivative
  Simulink-PS Converter : nesl_utility/Simulink-PS Converter  PhysicalDomain=network_engine_domain  SubClassName=ps_input  LeftPortType=input  RightPortType=output  PseudoPeriodic=off  Frequencies=[]  NoiseDistribution=none  NoiseParameters=[]  Unit=1  AffineConversion=off  InputFiltering=derivs  SimscapeFilterOrder=1  InputFilterTimeConstant=0.001  UdotUserProvided=2
  Conn1 : PMIOPort  Port=1  Side=Right
  wires:
  Derivative1/1 -> Simulink-PS Converter/3
  Derivative/1 -> Simulink-PS Converter/2, Derivative1/1
  In1/1 -> Derivative/1, Simulink-PS Converter/1
  connections:
  Simulink-PS Converter/RConn1 -- Conn1/RConn1

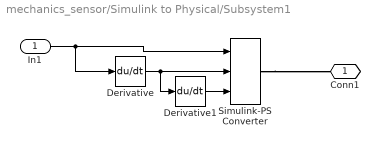
== system mechanics_sensor/Simulink to Physical/Subsystem1 ==
  In1 : Inport
  Derivative : Derivative
  Derivative1 : Derivative
  Simulink-PS Converter : nesl_utility/Simulink-PS Converter  PhysicalDomain=network_engine_domain  SubClassName=ps_input  LeftPortType=input  RightPortType=output  PseudoPeriodic=off  Frequencies=[]  NoiseDistribution=none  NoiseParameters=[]  Unit=1  AffineConversion=off  InputFiltering=derivs  SimscapeFilterOrder=1  InputFilterTimeConstant=0.001  UdotUserProvided=2
  Conn1 : PMIOPort  Port=1  Side=Right
  wires:
  Derivative1/1 -> Simulink-PS Converter/3
  Derivative/1 -> Simulink-PS Converter/2, Derivative1/1
  In1/1 -> Derivative/1, Simulink-PS Converter/1
  connections:
  Simulink-PS Converter/RConn1 -- Conn1/RConn1

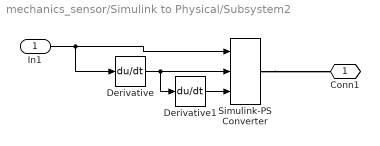
== system mechanics_sensor/Simulink to Physical/Subsystem2 ==
  In1 : Inport
  Derivative : Derivative
  Derivative1 : Derivative
  Simulink-PS Converter : nesl_utility/Simulink-PS Converter  PhysicalDomain=network_engine_domain  SubClassName=ps_input  LeftPortType=input  RightPortType=output  PseudoPeriodic=off  Frequencies=[]  NoiseDistribution=none  NoiseParameters=[]  Unit=1  AffineConversion=off  InputFiltering=derivs  SimscapeFilterOrder=1  InputFilterTimeConstant=0.001  UdotUserProvided=2
  Conn1 : PMIOPort  Port=1  Side=Right
  wires:
  Derivative1/1 -> Simulink-PS Converter/3
  Derivative/1 -> Simulink-PS Converter/2, Derivative1/1
  In1/1 -> Derivative/1, Simulink-PS Converter/1
  connections:
  Simulink-PS Converter/RConn1 -- Conn1/RConn1

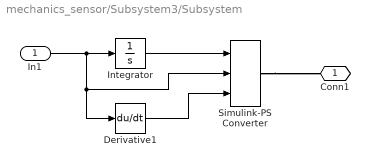
== system mechanics_sensor/Subsystem3/Subsystem ==
  In1 : Inport
  Derivative1 : Derivative
  Integrator : Integrator
  Simulink-PS Converter : nesl_utility/Simulink-PS Converter  PhysicalDomain=network_engine_domain  SubClassName=ps_input  LeftPortType=input  RightPortType=output  PseudoPeriodic=off  Frequencies=[]  NoiseDistribution=none  NoiseParameters=[]  Unit=1  AffineConversion=off  InputFiltering=derivs  SimscapeFilterOrder=1  InputFilterTimeConstant=0.001  UdotUserProvided=2
  Conn1 : PMIOPort  Port=1  Side=Right
  wires:
  Derivative1/1 -> Simulink-PS Converter/3
  In1/1 -> Simulink-PS Converter/2, Derivative1/1, Integrator/1
  Integrator/1 -> Simulink-PS Converter/1
  connections:
  Simulink-PS Converter/RConn1 -- Conn1/RConn1

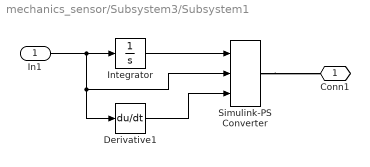
== system mechanics_sensor/Subsystem3/Subsystem1 ==
  In1 : Inport
  Derivative1 : Derivative
  Integrator : Integrator
  Simulink-PS Converter : nesl_utility/Simulink-PS Converter  PhysicalDomain=network_engine_domain  SubClassName=ps_input  LeftPortType=input  RightPortType=output  PseudoPeriodic=off  Frequencies=[]  NoiseDistribution=none  NoiseParameters=[]  Unit=1  AffineConversion=off  InputFiltering=derivs  SimscapeFilterOrder=1  InputFilterTimeConstant=0.001  UdotUserProvided=2
  Conn1 : PMIOPort  Port=1  Side=Right
  wires:
  Derivative1/1 -> Simulink-PS Converter/3
  In1/1 -> Simulink-PS Converter/2, Derivative1/1, Integrator/1
  Integrator/1 -> Simulink-PS Converter/1
  connections:
  Simulink-PS Converter/RConn1 -- Conn1/RConn1

== system mechanics_sensor/Subsystem3/Subsystem2 ==
  In1 : Inport
  Derivative1 : Derivative
  Integrator : Integrator
  Simulink-PS Converter : nesl_utility/Simulink-PS Converter  PhysicalDomain=network_engine_domain  SubClassName=ps_input  LeftPortType=input  RightPortType=output  PseudoPeriodic=off  Frequencies=[]  NoiseDistribution=none  NoiseParameters=[]  Unit=1  AffineConversion=off  InputFiltering=derivs  SimscapeFilterOrder=1  InputFilterTimeConstant=0.001  UdotUserProvided=2
  Conn1 : PMIOPort  Port=1  Side=Right
  wires:
  Derivative1/1 -> Simulink-PS Converter/3
  In1/1 -> Simulink-PS Converter/2, Derivative1/1, Integrator/1
  Integrator/1 -> Simulink-PS Converter/1
  connections:
  Simulink-PS Converter/RConn1 -- Conn1/RConn1
